simulink model "gyro"  (R2021b)
settings: Solver=VariableStepAuto  StartTime=0.0  StopTime=10.0  RelTol=1e-3
undefined symbols (not defined in the file): I_r, k, w_r
settings Model: Creator=jorgemarrero  LastModifiedBy=jorgemarrero

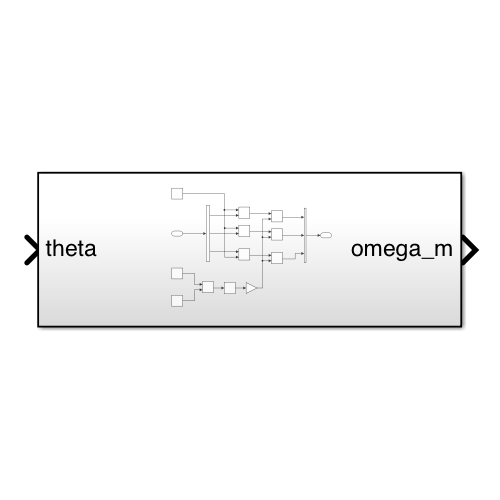
[thumbnail: Simulink's stored preview of the top-level diagram]
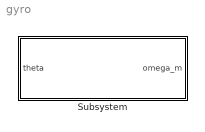
== system gyro ==
  Subsystem : Subsystem

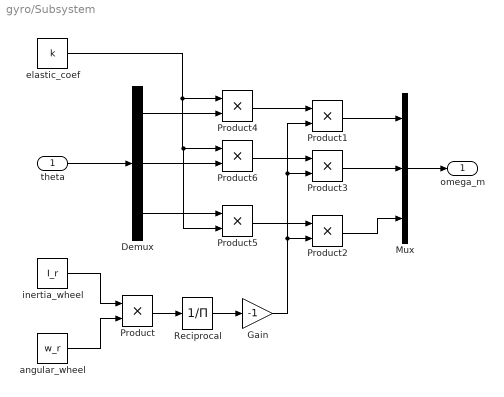
== system gyro/Subsystem ==
  theta : Inport
  Demux : Demux  Outputs=3
  Gain : Gain  Gain=-1
  Mux : Mux  Inputs=3
  Product{,1..6} (7 alike) : Product
  Reciprocal : Product  Inputs=/
  angular_wheel : Constant  Value=w_r
  "elastic_coef " : Constant  Value=k
  inertia_wheel : Constant  Value=I_r
  omega_m : Outport
  wires:
  Mux/1 -> omega_m/1
  Product4/1 -> Product1/1
  Product1/1 -> Mux/1
  inertia_wheel/1 -> Product/1
  Product6/1 -> Product3/1
  angular_wheel/1 -> Product/2
  Product/1 -> Reciprocal/1
  Demux/3 -> Product5/1
  Demux/2 -> Product6/2
  theta/1 -> Demux/1
  Reciprocal/1 -> Gain/1
  Demux/1 -> Product4/2
  Product3/1 -> Mux/2
  Product2/1 -> Mux/3
  Product5/1 -> Product2/1
  Gain/1 -> Product1/2, Product3/2, Product2/2
  "elastic_coef "/1 -> Product5/2, Product6/1, Product4/1
